simulink model "problem1_2_3"  (R2014b)
settings: Solver=ode3  StartTime=0.0  StopTime=41  FixedStep=0.01  RelTol=1e-3
InitFcn:
  | m_0 = 4000;
  | K = -3000;
  | t_0 = 36;
  | m_dot_initial = -35;
  | d = 0.17;
  | S =  pi * 0.25 * d^2;
  | rou_0 = 1.2251;
  | sigma = 7 * 10^(-6);
  | c_d = 0.4;
  | k  =  6371*10^3;
  | g_0 =  9.8;
  | T = K *m_dot_initial;
  | h = 1.271 * 10^4 ;
  | V = 771.7 ;
  | a = 27.46 ;
  | D_coef = 0.5 * rou_0 * S * c_d ;
  | Gravity_coef = g_0 * k^2 ;
  | Dr_coef = 0.5 * rou_0 * S * c_d ;
  | Dr_lin = V^2 * (1 - sigma * h);
  | m_lin = m_0 + m_dot_initial * t_0 ;
settings Model: Creator=mohsen  LastModifiedBy=SONY
settings DataIOCC: SignalLoggingSaveFormat=ModelDataLogs
settings DebuggingCC: UnderspecifiedInitializationDetection=Classic  MergeDetectMultiDrivingBlocksExec=none  MultiTaskDSMMsg=warning  MultiTaskCondExecSysMsg=none  StateNameClashWarn=warning  StrictBusMsg=None
settings RTWCC: IncludeERTFirstTime=on

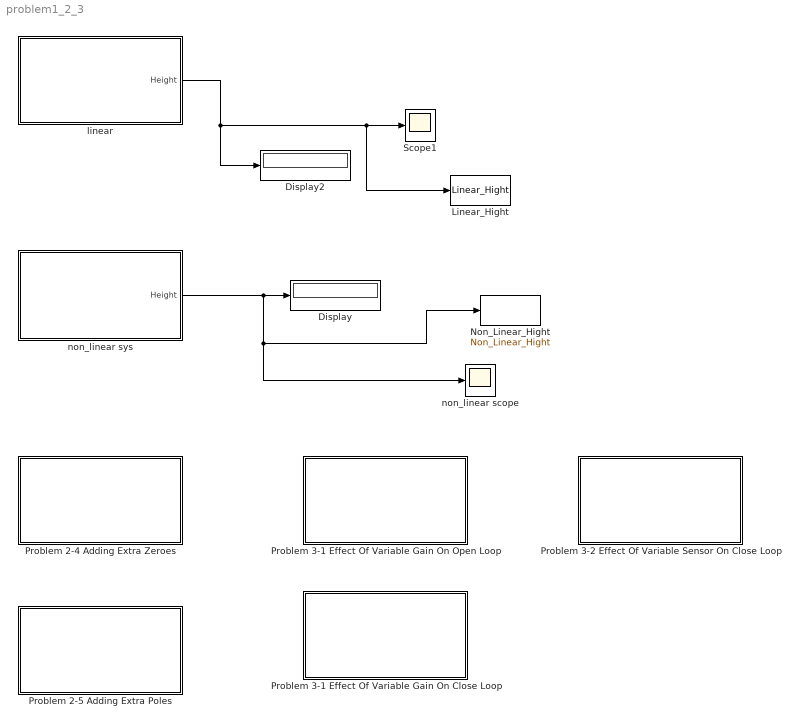
== system problem1_2_3 ==
  Display : Display
  Display2 : Display
  Linear_Hight : ToWorkspace  VariableName=Linear_Hight  SampleTime=-1
  Non_Linear_Hight : ToWorkspace  VariableName=Non_Linear_Hight  SampleTime=-1
  Problem 2-4 Adding Extra Zeroes : Subsystem
  Problem 2-5 Adding Extra Poles : Subsystem
  Problem 3-1 Effect Of Variable Gain On Close Loop : Subsystem
  Problem 3-1 Effect Of Variable Gain On Open Loop : Subsystem
  Problem 3-2 Effect Of Variable Sensor On Close Loop : Subsystem
  Scope1 : Scope
  linear : Subsystem
  non_linear scope : Scope
  non_linear sys : Subsystem
  wires:
  non_linear sys/1(Height) -> Non_Linear_Hight/1, non_linear scope/1, Display/1
  linear/1(Height) -> Linear_Hight/1, Scope1/1, Display2/1

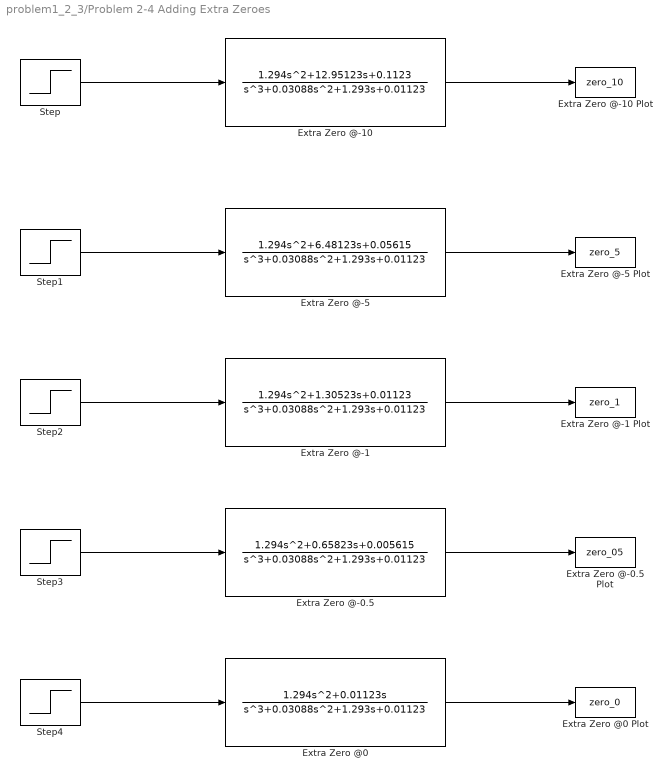
== system problem1_2_3/Problem 2-4 Adding Extra Zeroes ==
  Extra Zero @-0.5 : TransferFcn  Numerator=[1.294 0.65823 0.005615]  Denominator=[1 0.03088 1.293 0.01123]
  Extra Zero @-0.5 Plot : ToWorkspace  VariableName=zero_05  SampleTime=-1
  Extra Zero @-1 : TransferFcn  Numerator=[1.294 1.30523 0.01123]  Denominator=[1 0.03088 1.293 0.01123]
  Extra Zero @-1 Plot : ToWorkspace  VariableName=zero_1  SampleTime=-1
  Extra Zero @-10 : TransferFcn  Numerator=[1.294 12.95123 0.1123]  Denominator=[1 0.03088 1.293 0.01123]
  Extra Zero @-10 Plot : ToWorkspace  VariableName=zero_10  SampleTime=-1
  Extra Zero @-5 : TransferFcn  Numerator=[1.294 6.48123 0.05615]  Denominator=[1 0.03088 1.293 0.01123]
  Extra Zero @-5 Plot : ToWorkspace  VariableName=zero_5  SampleTime=-1
  Extra Zero @0 : TransferFcn  Numerator=[1.294 0.01123 0]  Denominator=[1 0.03088 1.293 0.01123]
  Extra Zero @0 Plot : ToWorkspace  VariableName=zero_0  SampleTime=-1
  Step{,1..4} (5 alike) : Step  SampleTime=0
  wires:
  Step/1 -> Extra Zero @-10/1
  Extra Zero @-10/1 -> Extra Zero @-10 Plot/1
  Step1/1 -> Extra Zero @-5/1
  Extra Zero @-5/1 -> Extra Zero @-5 Plot/1
  Step2/1 -> Extra Zero @-1/1
  Extra Zero @-1/1 -> Extra Zero @-1 Plot/1
  Step3/1 -> Extra Zero @-0.5/1
  Extra Zero @-0.5/1 -> Extra Zero @-0.5 Plot/1
  Step4/1 -> Extra Zero @0/1
  Extra Zero @0/1 -> Extra Zero @0 Plot/1

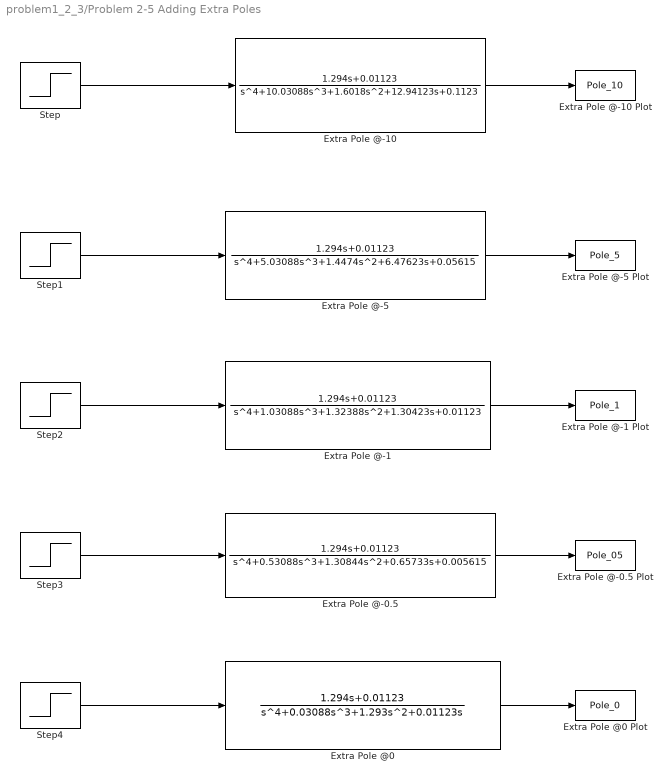
== system problem1_2_3/Problem 2-5 Adding Extra Poles ==
  Extra Pole @-0.5 : TransferFcn  Numerator=[1.294 0.01123]  Denominator=[1 0.53088 1.30844 0.65733 0.005615]
  Extra Pole @-0.5 Plot : ToWorkspace  VariableName=Pole_05  SampleTime=-1
  Extra Pole @-1 : TransferFcn  Numerator=[1.294 0.01123]  Denominator=[1 1.03088 1.32388 1.30423 0.01123]
  Extra Pole @-1 Plot : ToWorkspace  VariableName=Pole_1  SampleTime=-1
  Extra Pole @-10 : TransferFcn  Numerator=[1.294 0.01123]  Denominator=[1 10.03088 1.6018 12.94123 0.1123]
  Extra Pole @-10 Plot : ToWorkspace  VariableName=Pole_10  SampleTime=-1
  Extra Pole @-5 : TransferFcn  Numerator=[1.294 0.01123]  Denominator=[1 5.03088 1.4474 6.47623 0.05615]
  Extra Pole @-5 Plot : ToWorkspace  VariableName=Pole_5  SampleTime=-1
  Extra Pole @0 : TransferFcn  Numerator=[1.294 0.01123]  Denominator=[1 0.03088 1.293 0.01123 0]
  Extra Pole @0 Plot : ToWorkspace  VariableName=Pole_0  SampleTime=-1
  Step{,1..4} (5 alike) : Step  SampleTime=0
  wires:
  Step/1 -> Extra Pole @-10/1
  Extra Pole @-10/1 -> Extra Pole @-10 Plot/1
  Step1/1 -> Extra Pole @-5/1
  Extra Pole @-5/1 -> Extra Pole @-5 Plot/1
  Step2/1 -> Extra Pole @-1/1
  Extra Pole @-1/1 -> Extra Pole @-1 Plot/1
  Step3/1 -> Extra Pole @-0.5/1
  Extra Pole @-0.5/1 -> Extra Pole @-0.5 Plot/1
  Step4/1 -> Extra Pole @0/1
  Extra Pole @0/1 -> Extra Pole @0 Plot/1

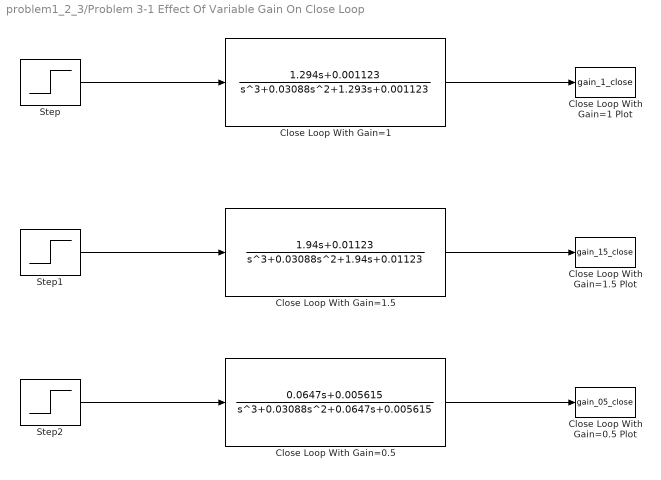
== system problem1_2_3/Problem 3-1 Effect Of Variable Gain On Close Loop ==
  Close Loop With Gain=0.5 : TransferFcn  Numerator=[0.0647 0.005615]  Denominator=[1 0.03088 0.0647 0.005615]
  Close Loop With Gain=0.5 Plot : ToWorkspace  VariableName=gain_05_close  SampleTime=-1
  Close Loop With Gain=1 : TransferFcn  Numerator=[1.294 0.001123 ]  Denominator=[1 0.03088 1.293 0.001123]
  Close Loop With Gain=1 Plot : ToWorkspace  VariableName=gain_1_close  SampleTime=-1
  Close Loop With Gain=1.5 : TransferFcn  Numerator=[1.94 0.01123]  Denominator=[1 0.03088 1.94 0.01123]
  Close Loop With Gain=1.5 Plot : ToWorkspace  VariableName=gain_15_close  SampleTime=-1
  Step : Step  SampleTime=0
  Step1 : Step  SampleTime=0
  Step2 : Step  SampleTime=0
  wires:
  Step/1 -> Close Loop With Gain=1/1
  Close Loop With Gain=1/1 -> Close Loop With Gain=1 Plot/1
  Step1/1 -> Close Loop With Gain=1.5/1
  Close Loop With Gain=1.5/1 -> Close Loop With Gain=1.5 Plot/1
  Step2/1 -> Close Loop With Gain=0.5/1
  Close Loop With Gain=0.5/1 -> Close Loop With Gain=0.5 Plot/1

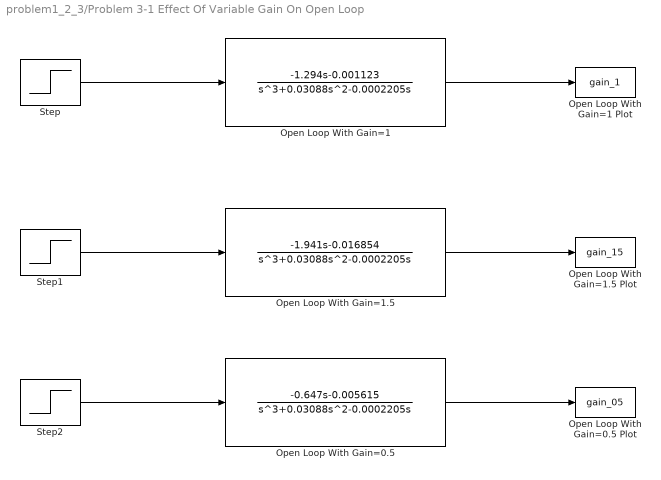
== system problem1_2_3/Problem 3-1 Effect Of Variable Gain On Open Loop ==
  Open Loop With Gain=0.5 : TransferFcn  Numerator=[-0.647 -0.005615]  Denominator=[1 0.03088 -0.0002205 0]
  Open Loop With Gain=0.5 Plot : ToWorkspace  VariableName=gain_05  SampleTime=-1
  Open Loop With Gain=1 : TransferFcn  Numerator=[-1.294 -0.001123 ]  Denominator=[1 0.03088 -0.0002205 0]
  Open Loop With Gain=1 Plot : ToWorkspace  VariableName=gain_1  SampleTime=-1
  Open Loop With Gain=1.5 : TransferFcn  Numerator=[-1.941 -0.016854]  Denominator=[1 0.03088 -0.0002205 0]
  Open Loop With Gain=1.5 Plot : ToWorkspace  VariableName=gain_15  SampleTime=-1
  Step : Step  After=-41  SampleTime=0
  Step1 : Step  After=-41  SampleTime=0
  Step2 : Step  After=-41  SampleTime=0
  wires:
  Step/1 -> Open Loop With Gain=1/1
  Open Loop With Gain=1/1 -> Open Loop With Gain=1 Plot/1
  Step1/1 -> Open Loop With Gain=1.5/1
  Open Loop With Gain=1.5/1 -> Open Loop With Gain=1.5 Plot/1
  Step2/1 -> Open Loop With Gain=0.5/1
  Open Loop With Gain=0.5/1 -> Open Loop With Gain=0.5 Plot/1

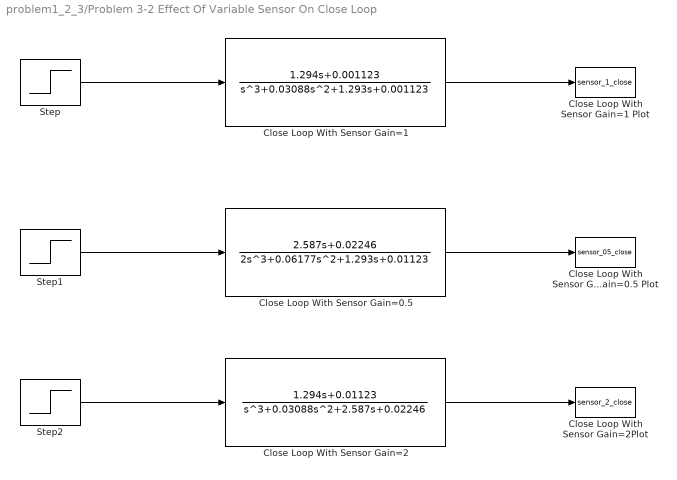
== system problem1_2_3/Problem 3-2 Effect Of Variable Sensor On Close Loop ==
  Close Loop With Sensor Gain=0.5 : TransferFcn  Numerator=[2.587 0.02246]  Denominator=[2 0.06177 1.293 0.01123]
  Close Loop With Sensor Gain=0.5 Plot : ToWorkspace  VariableName=sensor_05_close  SampleTime=-1
  Close Loop With Sensor Gain=1 : TransferFcn  Numerator=[1.294 0.001123 ]  Denominator=[1 0.03088 1.293 0.001123]
  Close Loop With Sensor Gain=1 Plot : ToWorkspace  VariableName=sensor_1_close  SampleTime=-1
  Close Loop With Sensor Gain=2 : TransferFcn  Numerator=[1.294 0.01123]  Denominator=[1 0.03088 2.587 0.02246]
  Close Loop With Sensor Gain=2Plot : ToWorkspace  VariableName=sensor_2_close  SampleTime=-1
  Step : Step  SampleTime=0
  Step1 : Step  SampleTime=0
  Step2 : Step  SampleTime=0
  wires:
  Step/1 -> Close Loop With Sensor Gain=1/1
  Close Loop With Sensor Gain=1/1 -> Close Loop With Sensor Gain=1 Plot/1
  Step1/1 -> Close Loop With Sensor Gain=0.5/1
  Close Loop With Sensor Gain=0.5/1 -> Close Loop With Sensor Gain=0.5 Plot/1
  Step2/1 -> Close Loop With Sensor Gain=2/1
  Close Loop With Sensor Gain=2/1 -> Close Loop With Sensor Gain=2Plot/1

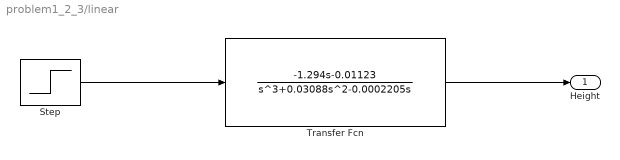
== system problem1_2_3/linear ==
  Step : Step  After=-41  SampleTime=0
  Transfer Fcn : TransferFcn  Numerator=[-1.294 -0.01123]  Denominator=[1 0.03088 -0.0002205 0]
  Height : Outport
  wires:
  Step/1 -> Transfer Fcn/1
  Transfer Fcn/1 -> Height/1

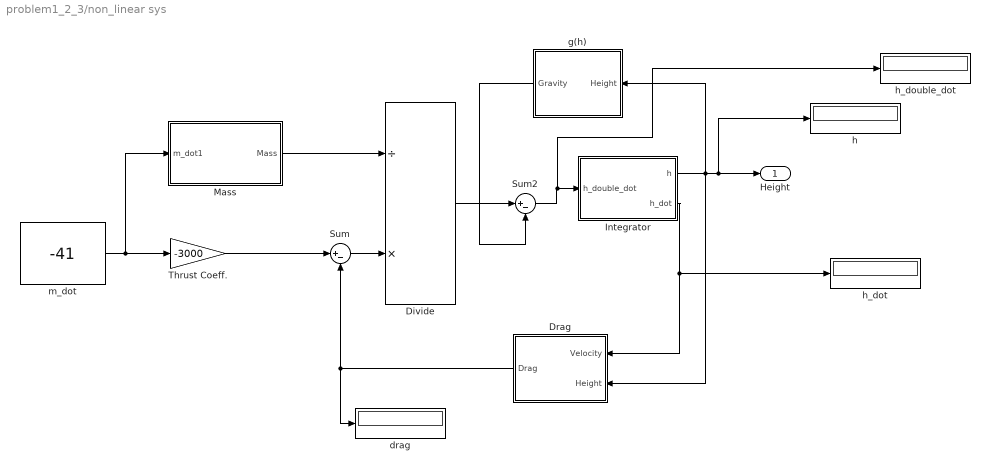
== system problem1_2_3/non_linear sys ==
  Divide : Product  Inputs=/*
  Drag : Subsystem
  Integrator : Subsystem
  Mass : Subsystem
  Sum : Sum  Inputs=|+-
  Sum2 : Sum  Inputs=|+-
  Thrust Coeff. : Gain  Gain=-3000
  drag : Display
  g(h) : Subsystem
  h : Display
  h_dot : Display
  h_double_dot : Display
  m_dot : Constant  Value=-41
  Height : Outport
  wires:
  Integrator/2(h_dot) -> h_dot/1, Drag/1(Velocity)
  Drag/1(Drag) -> drag/1, Sum/2
  Mass/1(Mass) -> Divide/1
  m_dot/1 -> Mass/1(m_dot1), Thrust Coeff./1
  Sum2/1 -> h_double_dot/1, Integrator/1(h_double_dot)
  Sum/1 -> Divide/2
  Integrator/1(h) -> h/1, Height/1, Drag/2(Height), g(h)/1(Height)
  Thrust Coeff./1 -> Sum/1
  g(h)/1(Gravity) -> Sum2/2
  Divide/1 -> Sum2/1

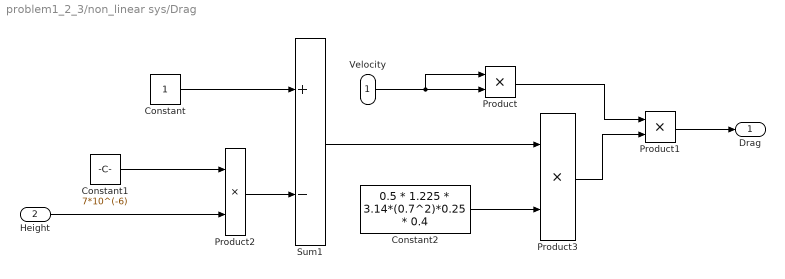
== system problem1_2_3/non_linear sys/Drag ==
  Velocity : Inport
  Height : Inport  Port=2
  Constant : Constant
  Constant1 : Constant  Value=7*10^(-6)
  Constant2 : Constant  Value=0.5 * 1.225 * 3.14*(0.7^2)*0.25 * 0.4
  Product{,1..3} (4 alike) : Product
  Sum1 : Sum  Inputs=+-
  Drag : Outport
  wires:
  Product1/1 -> Drag/1
  Height/1 -> Product2/2
  Constant/1 -> Sum1/1
  Product2/1 -> Sum1/2
  Product/1 -> Product1/1
  Sum1/1 -> Product3/1
  Constant1/1 -> Product2/1
  Velocity/1 -> Product/1, Product/2
  Constant2/1 -> Product3/2
  Product3/1 -> Product1/2

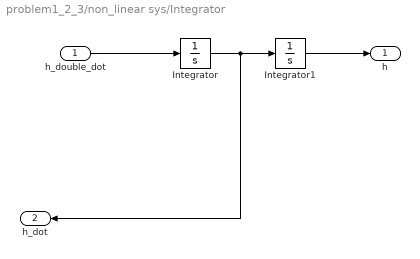
== system problem1_2_3/non_linear sys/Integrator ==
  h_double_dot : Inport
  Integrator : Integrator
  Integrator1 : Integrator
  h : Outport
  h_dot : Outport  Port=2
  wires:
  h_double_dot/1 -> Integrator/1
  Integrator1/1 -> h/1
  Integrator/1 -> h_dot/1, Integrator1/1

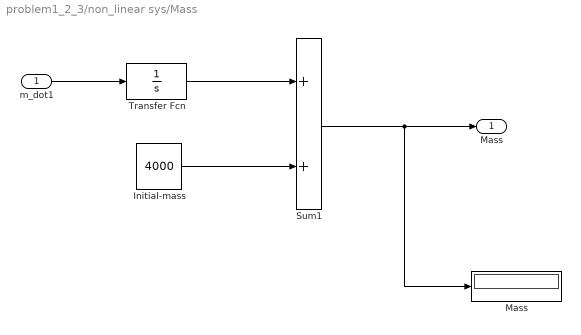
== system problem1_2_3/non_linear sys/Mass ==
  m_dot1 : Inport
  Initial-mass : Constant  Value=4000
  "Mass " : Display
  Sum1 : Sum
  Transfer Fcn : TransferFcn  Denominator=[1 0]
  Mass : Outport
  wires:
  m_dot1/1 -> Transfer Fcn/1
  Initial-mass/1 -> Sum1/2
  Sum1/1 -> "Mass "/1, Mass/1
  Transfer Fcn/1 -> Sum1/1

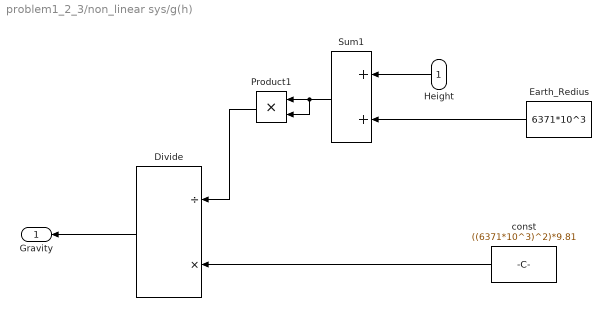
== system problem1_2_3/non_linear sys/g(h) ==
  Height : Inport
  Divide : Product  Inputs=/*
  Earth_Redius : Constant  Value=6371*10^3
  Product1 : Product
  Sum1 : Sum
  const : Constant  Value=((6371*10^3)^2)*9.81
  Gravity : Outport
  wires:
  Height/1 -> Sum1/1
  Earth_Redius/1 -> Sum1/2
  Sum1/1 -> Product1/2, Product1/1
  Product1/1 -> Divide/1
  Divide/1 -> Gravity/1
  const/1 -> Divide/2
